simulink library "SAD"  (R2025b)
settings: Solver=VariableStepAuto  StartTime=0.0  StopTime=10.0  RelTol=1e-3
values from neighbouring files (symbols this model uses):
  c = astroConstants(5)*10^3    [RUN_ME.m]
  D = zeros(3)    [RUN_ME.m]
  Fe = 1358    [RUN_ME.m]
  I = [Ix 0 0; 0 Iy 0; 0 0 Iz]    [RUN_ME.m]
  Ix = (m_b/12)*((y_b^2)+(x_b^2))    (= 0.13)    [RUN_ME.m]
  Iy = (m_b/12)*((z_b^2)+(x_b^2))    (= 0.1)    [RUN_ME.m]
  Iz = (m_b/12)*((y_b^2)+(z_b^2))    (= 0.05)    [RUN_ME.m]
  n = sqrt(mu/a^3)    [RUN_ME.m]
  Ts = 0.1    [RUN_ME.m]
undefined symbols (not defined in the file or in its folder): A0, att0, Ir, Noise_pwr, Noise_st, omega_act_0, q0, RW_max_slope, RW_max_torque, RW_max_torque_descending_rate, RW_max_torque_start_descending, RW_min_torque, RW_offset, RW_tau_m, Satellite, w0, wr0
libraries: matrix_library x5, simulink x2, dspmathops x1
settings Model: Creator=ludod  LastModifiedBy=stefa

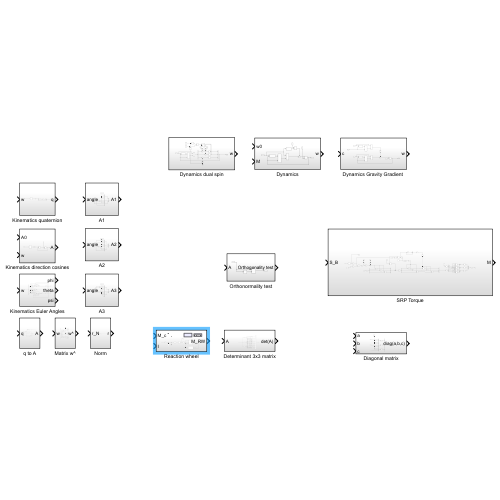
[thumbnail: Simulink's stored preview of the top-level diagram]
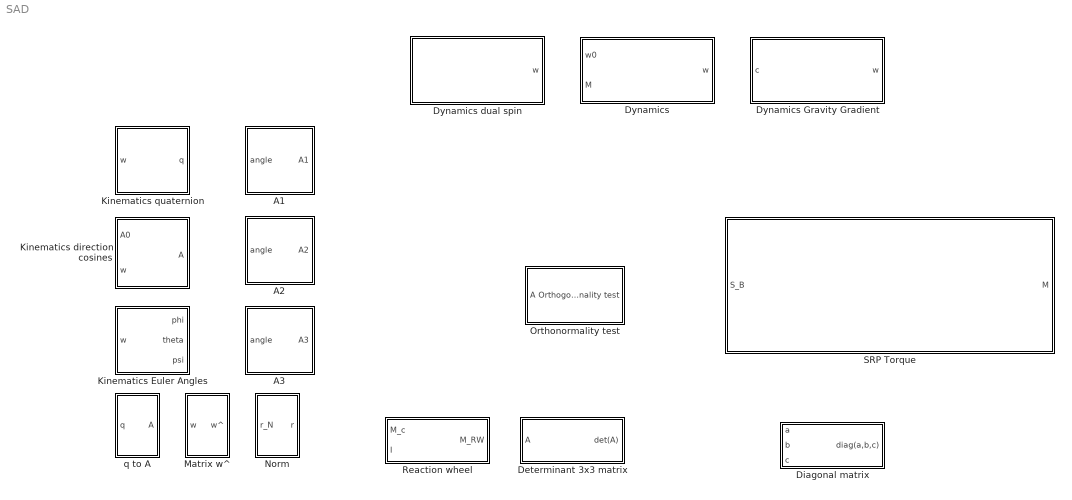
== system SAD ==
  A1 : Subsystem
  A2 : Subsystem
  A3 : Subsystem
  Determinant 3x3 matrix : Subsystem
  Diagonal matrix : Subsystem
  Dynamics : Subsystem
  "Dynamics Gravity Gradient " : Subsystem
  Dynamics dual spin : Subsystem
  Kinematics Euler Angles : Subsystem
  Kinematics direction cosines : Subsystem
  Kinematics quaternion : Subsystem
  Matrix w^ : Subsystem
  Norm : Subsystem
  Orthonormality test : Subsystem
  Reaction wheel : Subsystem
  SRP Torque : Subsystem
  q to A : Subsystem

== system SAD/A1 ==
  angle : Inport
  Cos : Trigonometry  Operator=cos
  Gain : Gain  Gain=-1
  Mux : Mux  Inputs=3
  Mux1 : Mux  Inputs=3
  Mux2 : Mux  Inputs=3
  One : Constant  OutDataTypeStr=Inherit: Inherit via back propagation
  Sin : Trigonometry
  Vector Concatenate : Concatenate  NumInputs=3  Mode=Multidimensional array  ConcatenateDimension=2
  Zero : Constant  Value=0  OutDataTypeStr=Inherit: Inherit via back propagation
  A1 : Outport
  wires:
  Zero/1 -> Mux2/1, Mux1/1, Mux/3, Mux/2
  One/1 -> Mux/1
  Sin/1 -> Mux2/2, Gain/1
  angle/1 -> Sin/1, Cos/1
  Vector Concatenate/1 -> A1/1  "A1"
  Gain/1 -> Mux1/3
  Cos/1 -> Mux2/3, Mux1/2
  Mux/1 -> Vector Concatenate/1
  Mux1/1 -> Vector Concatenate/2
  Mux2/1 -> Vector Concatenate/3

== system SAD/A2 ==
  angle : Inport
  Cos : Trigonometry  Operator=cos
  Gain : Gain  Gain=-1
  Mux : Mux  Inputs=3
  Mux1 : Mux  Inputs=3
  Mux2 : Mux  Inputs=3
  One : Constant  OutDataTypeStr=Inherit: Inherit via back propagation
  Sin : Trigonometry
  Vector Concatenate : Concatenate  NumInputs=3  Mode=Multidimensional array  ConcatenateDimension=2
  Zero : Constant  Value=0  OutDataTypeStr=Inherit: Inherit via back propagation
  A2 : Outport
  wires:
  Mux1/1 -> Vector Concatenate/2
  Mux2/1 -> Vector Concatenate/3
  Zero/1 -> Mux2/2, Mux1/3, Mux1/1, Mux/2
  One/1 -> Mux1/2
  Mux/1 -> Vector Concatenate/1
  Sin/1 -> Mux/3, Gain/1
  angle/1 -> Sin/1, Cos/1
  Vector Concatenate/1 -> A2/1  "A2"
  Cos/1 -> Mux2/3, Mux/1
  Gain/1 -> Mux2/1

== system SAD/A3 ==
  angle : Inport
  Cos : Trigonometry  Operator=cos
  Gain : Gain  Gain=-1
  Mux : Mux  Inputs=3
  Mux1 : Mux  Inputs=3
  Mux2 : Mux  Inputs=3
  One : Constant  OutDataTypeStr=Inherit: Inherit via back propagation
  Sin : Trigonometry
  Vector Concatenate : Concatenate  NumInputs=3  Mode=Multidimensional array  ConcatenateDimension=2
  Zero : Constant  Value=0  OutDataTypeStr=Inherit: Inherit via back propagation
  A3 : Outport
  wires:
  Mux1/1 -> Vector Concatenate/2
  Mux2/1 -> Vector Concatenate/3
  Zero/1 -> Mux1/3, Mux2/2, Mux2/1, Mux/3
  Mux/1 -> Vector Concatenate/1
  Sin/1 -> Mux1/1, Gain/1
  angle/1 -> Sin/1, Cos/1
  Vector Concatenate/1 -> A3/1  "A3"
  Cos/1 -> Mux1/2, Mux/1
  Gain/1 -> Mux/2
  One/1 -> Mux2/3

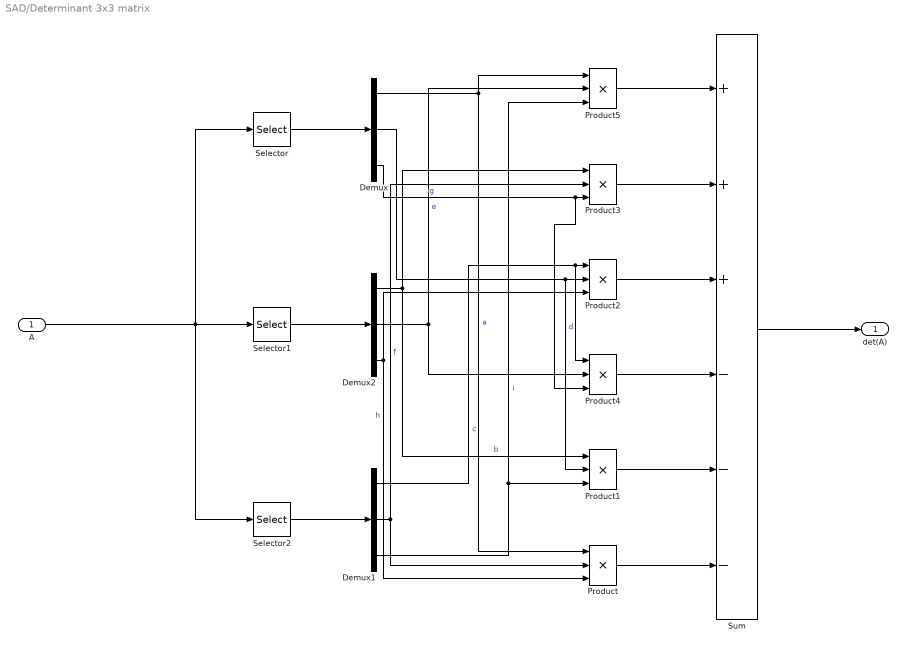
== system SAD/Determinant 3x3 matrix ==
  A : Inport
  Demux : Demux  Outputs=3
  Demux1 : Demux  Outputs=3
  Demux2 : Demux  Outputs=3
  Product{,1..5} (6 alike) : Product  Inputs=3
  Selector : Selector  NumberOfDimensions=2  InputPortWidth=3  IndexOptions=Index vector (dialog),Index vector (dialog)  Indices=1:3,1  OutputSizes=1,1
  Selector1 : Selector  NumberOfDimensions=2  InputPortWidth=3  IndexOptions=Index vector (dialog),Index vector (dialog)  Indices=1:3,2  OutputSizes=1,1
  Selector2 : Selector  NumberOfDimensions=2  InputPortWidth=3  IndexOptions=Index vector (dialog),Index vector (dialog)  Indices=1:3,3  OutputSizes=1,1
  Sum : Sum  Inputs=+++---
  det(A) : Outport
  wires:
  A/1 -> Selector1/1, Selector/1, Selector2/1
  Selector/1 -> Demux/1
  Selector1/1 -> Demux2/1
  Selector2/1 -> Demux1/1
  Demux/1 -> Product/1, Product5/1  "a"
  Demux/2 -> Product2/2, Product1/2  "d"
  Demux/3 -> Product4/3, Product3/3  "g"
  Demux2/1 -> Product1/1, Product3/1  "b"
  Demux2/2 -> Product4/2, Product5/2  "e"
  Demux2/3 -> Product2/3, Product/3  "h"
  Demux1/1 -> Product4/1, Product2/1  "c"
  Demux1/2 -> Product/2, Product3/2  "f"
  Demux1/3 -> Product1/3, Product5/3  "i"
  Product/1 -> Sum/6
  Product1/1 -> Sum/5
  Product4/1 -> Sum/4
  Product2/1 -> Sum/3
  Product3/1 -> Sum/2
  Product5/1 -> Sum/1
  Sum/1 -> det(A)/1

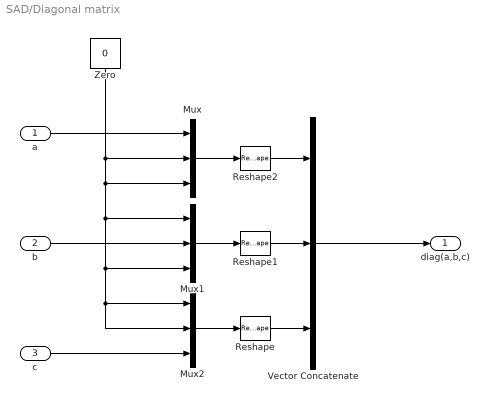
== system SAD/Diagonal matrix ==
  a : Inport
  b : Inport  Port=2
  c : Inport  Port=3
  Mux : Mux  Inputs=3
  Mux1 : Mux  Inputs=3
  Mux2 : Mux  Inputs=3
  Reshape : Reshape  OutputDimensionality=Column vector (2-D)
  Reshape1 : Reshape  OutputDimensionality=Column vector (2-D)
  Reshape2 : Reshape  OutputDimensionality=Column vector (2-D)
  Vector Concatenate : Concatenate  NumInputs=3  Mode=Multidimensional array  ConcatenateDimension=2
  Zero : Constant  Value=0  OutDataTypeStr=Inherit: Inherit via back propagation
  diag(a,b,c) : Outport
  wires:
  a/1 -> Mux/1
  b/1 -> Mux1/2
  c/1 -> Mux2/3
  Zero/1 -> Mux/2, Mux/3, Mux1/1, Mux1/3, Mux2/2, Mux2/1
  Mux/1 -> Reshape2/1
  Mux1/1 -> Reshape1/1
  Mux2/1 -> Reshape/1
  Vector Concatenate/1 -> diag(a,b,c)/1
  Reshape2/1 -> Vector Concatenate/1
  Reshape1/1 -> Vector Concatenate/2
  Reshape/1 -> Vector Concatenate/3

== system SAD/Dynamics ==
  w0 : Inport
  M : Inport  Port=2
  Constant : Constant  Value=I
  Cross Product : matrix_library/Cross Product
  Divide : Product  Inputs=*/
  Extract Diagonal : matrix_library/Extract Diagonal
      settings: LibrarySourceBlock=|
      | simulink/Matrix
      | Operations/Extract Diagonal
  Integrator : Integrator  InitialConditionSource=external
  Product : Product  Multiplication=Matrix(*)
  Product1 : Product  Inputs=/*  Multiplication=Matrix(*)
  Sum : Sum  Inputs=++|
  w : Outport
  wires:
  w0/1 -> Integrator/2
  Constant/1 -> Product1/1, Extract Diagonal/1, Product/1
  Integrator/1 -> w/1, Product/2, Cross Product/2
  Cross Product/1 -> Product1/2
  Product/1 -> Cross Product/1
  M/1 -> Divide/1
  Divide/1 -> Sum/1
  Product1/1 -> Sum/2
  Sum/1 -> Integrator/1
  Extract Diagonal/1 -> Divide/2

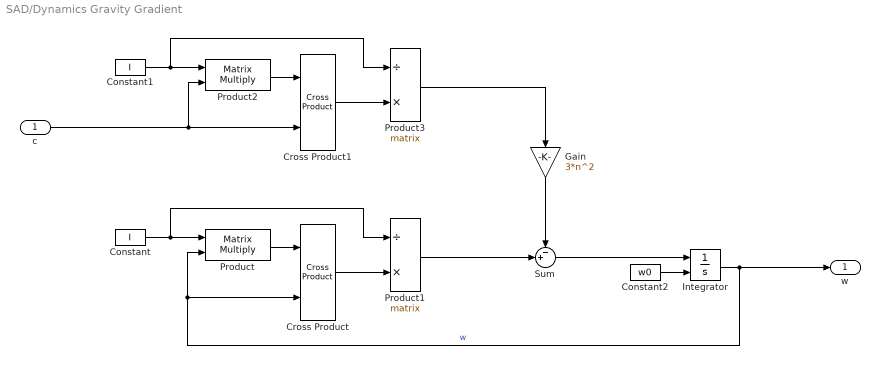
== system SAD/Dynamics Gravity Gradient  ==
  c : Inport
  Constant : Constant  Value=I
  Constant1 : Constant  Value=I
  Constant2 : Constant  Value=w0
  Cross Product : matrix_library/Cross Product
  Cross Product1 : matrix_library/Cross Product
  Gain : Gain  Gain=3*n^2
  Integrator : Integrator  InitialConditionSource=external
  Product : Product  Multiplication=Matrix(*)
  Product1 : Product  Inputs=/*  Multiplication=Matrix(*)
  Product2 : Product  Multiplication=Matrix(*)
  Product3 : Product  Inputs=/*  Multiplication=Matrix(*)
  Sum : Sum  Inputs=-+|
  w : Outport
  wires:
  Product/1 -> Cross Product/1
  Product2/1 -> Cross Product1/1
  Integrator/1 -> w/1, Cross Product/2, Product/2  "w"
  Product3/1 -> Gain/1
  c/1 -> Product2/2, Cross Product1/2
  Constant2/1 -> Integrator/2
  Constant1/1 -> Product3/1, Product2/1
  Cross Product/1 -> Product1/2
  Product1/1 -> Sum/2
  Sum/1 -> Integrator/1
  Constant/1 -> Product/1, Product1/1
  Gain/1 -> Sum/1
  Cross Product1/1 -> Product3/2

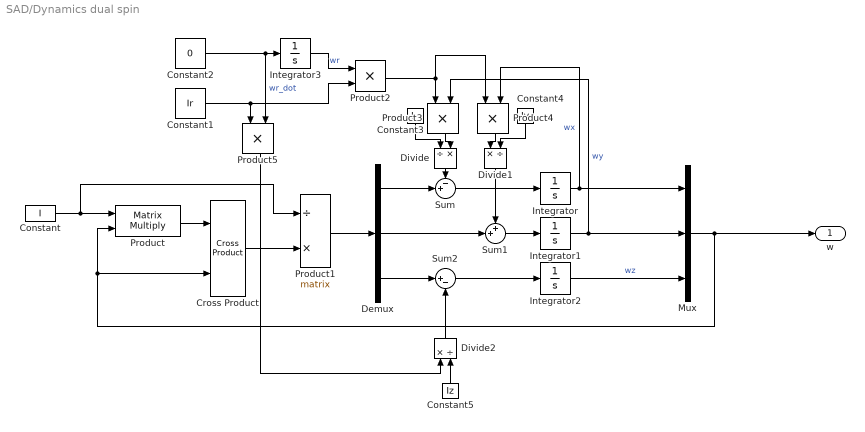
== system SAD/Dynamics dual spin ==
  Constant : Constant  Value=I
  Constant1 : Constant  Value=Ir
  Constant2 : Constant  Value=0
  Constant3 : Constant  Value=Ix
  Constant4 : Constant  Value=Iy
  Constant5 : Constant  Value=Iz
  Cross Product : matrix_library/Cross Product
  Demux : Demux  Outputs=3
  Divide : Product  Inputs=/*
  Divide1 : Product  Inputs=*/
  Divide2 : Product  Inputs=*/
  Integrator : Integrator  InitialCondition=w0(1)
  Integrator1 : Integrator  InitialCondition=w0(2)
  Integrator2 : Integrator  InitialCondition=w0(3)
  Integrator3 : Integrator  InitialCondition=wr0
  Mux : Mux  Inputs=3
  Product : Product  Multiplication=Matrix(*)
  Product1 : Product  Inputs=/*  Multiplication=Matrix(*)
  Product{2..5} (4 alike) : Product
  Sum : Sum  Inputs=-+|
  Sum1 : Sum  Inputs=++|
  Sum2 : Sum  Inputs=|+-
  w : Outport
  wires:
  Constant1/1 -> Product2/2, Product5/1
  Product5/1 -> Divide2/1
  Divide2/1 -> Sum2/2
  Integrator1/1 -> Mux/2, Product3/2  "wy"
  Demux/2 -> Sum1/2
  Cross Product/1 -> Product1/2
  Demux/3 -> Sum2/1
  Sum/1 -> Integrator/1
  Divide/1 -> Sum/1
  Constant/1 -> Product1/1, Product/1
  Mux/1 -> w/1, Product/2, Cross Product/2
  Constant4/1 -> Divide1/2
  Demux/1 -> Sum/2
  Sum1/1 -> Integrator1/1
  Integrator/1 -> Mux/1, Product4/2  "wx"
  Integrator2/1 -> Mux/3  "wz"
  Product/1 -> Cross Product/1
  Product4/1 -> Divide1/1
  Product2/1 -> Product4/1, Product3/1
  Constant3/1 -> Divide/1
  Constant2/1 -> Product5/2, Integrator3/1  "wr_dot"
  Product3/1 -> Divide/2
  Product1/1 -> Demux/1
  Constant5/1 -> Divide2/2
  Integrator3/1 -> Product2/1  "wr"
  Sum2/1 -> Integrator2/1
  Divide1/1 -> Sum1/1

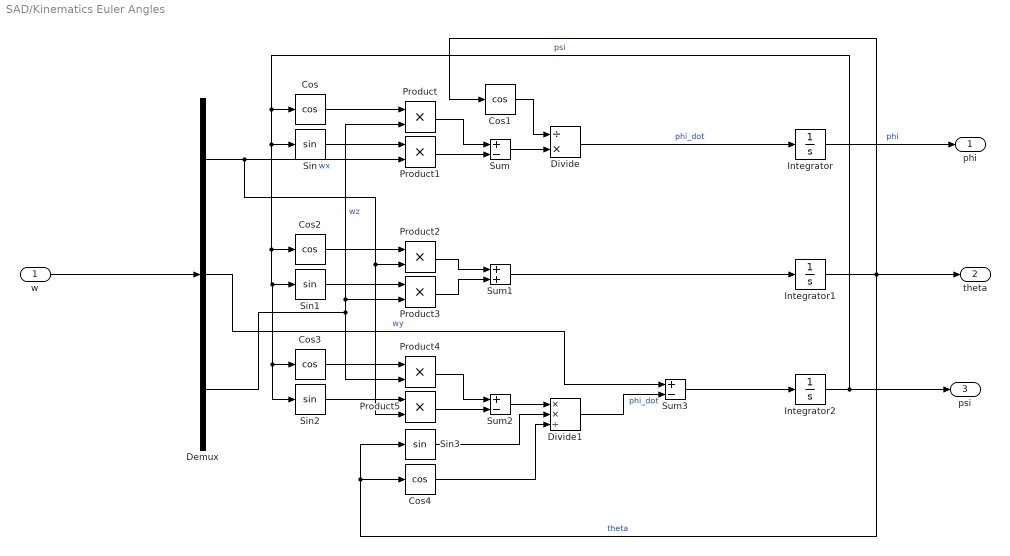
== system SAD/Kinematics Euler Angles ==
  w : Inport
  Cos{,1..4} (5 alike) : Trigonometry  Operator=cos
  Demux : Demux  Outputs=3
  Divide : Product  Inputs=/*
  Divide1 : Product  Inputs=**/
  Integrator : Integrator  InitialCondition=att0(1)  WrapState=on
  Integrator1 : Integrator  InitialCondition=att0(2)  WrapState=on
  Integrator2 : Integrator  InitialCondition=att0(3)  WrapState=on
  Product{,1..5} (6 alike) : Product
  Sin{,1..3} (4 alike) : Trigonometry
  Sum : Sum  Inputs=+-
  Sum1 : Sum
  Sum2 : Sum  Inputs=+-
  Sum3 : Sum  Inputs=+-
  phi : Outport
  theta : Outport  Port=2
  psi : Outport  Port=3
  wires:
  Cos1/1 -> Divide/1
  Demux/3 -> Product4/2, Product3/2, Product/2  "wz"
  Sin3/1 -> Divide1/2
  Product2/1 -> Sum1/1
  Product/1 -> Sum/1
  Integrator2/1 -> psi/1, Sin2/1, Cos3/1, Sin1/1, Cos2/1, Sin/1, Cos/1  "psi"
  Sin1/1 -> Product3/1
  Sin/1 -> Product1/1
  Integrator1/1 -> theta/1, Cos4/1, Sin3/1, Cos1/1  "theta"
  Cos2/1 -> Product2/1
  Cos/1 -> Product/1
  Sum1/1 -> Integrator1/1
  Cos3/1 -> Product4/1
  Demux/1 -> Product1/2, Product5/2, Product2/2  "wx"
  Integrator/1 -> phi/1  "phi"
  Product4/1 -> Sum2/1
  Sin2/1 -> Product5/1
  Product3/1 -> Sum1/2
  Demux/2 -> Sum3/1  "wy"
  Product1/1 -> Sum/2
  Sum/1 -> Divide/2
  Divide/1 -> Integrator/1  "phi_dot"
  Product5/1 -> Sum2/2
  Sum2/1 -> Divide1/1
  w/1 -> Demux/1
  Sum3/1 -> Integrator2/1
  Divide1/1 -> Sum3/2  "phi_dot"
  Cos4/1 -> Divide1/3

== system SAD/Kinematics direction cosines ==
  A0 : Inport
  w : Inport  Port=2
  Gain : Gain  Gain=-1
  Integrator : Integrator  InitialConditionSource=external  InitialCondition=A0
  Matrix w^ : Subsystem
  Product1 : Product  Multiplication=Matrix(*)
  A : Outport
  wires:
  Product1/1 -> Integrator/1  "A_dot"
  Matrix w^/1(w^) -> Gain/1  "w^"
  Integrator/1 -> A/1, Product1/2  "A"
  Gain/1 -> Product1/1
  w/1 -> Matrix w^/1(w)
  A0/1 -> Integrator/2

== system SAD/Kinematics quaternion ==
  w : Inport
  Gain : Gain  Gain=1/2
  Integrator1 : Integrator  InitialCondition=q0
  Omega matrix : Subsystem
  Product : Product  Multiplication=Matrix(*)
  Reshape : Reshape  OutputDimensionality=Column vector (2-D)
  q : Outport
  wires:
  Reshape/1 -> q/1, Product/2
  Integrator1/1 -> Reshape/1  "q"
  Omega matrix/1(Omega) -> Gain/1
  w/1 -> Omega matrix/1(w)
  Product/1 -> Integrator1/1  "q_dot"
  Gain/1 -> Product/1

== system SAD/Matrix w^ ==
  w : Inport
  Demux1 : Demux  Outputs=3
  Gain : Gain  Gain=-1
  Gain3 : Gain  Gain=-1
  Gain5 : Gain  Gain=-1
  Mux : Mux  Inputs=3
  Mux1 : Mux  Inputs=3
  Mux2 : Mux  Inputs=3
  Vector Concatenate : Concatenate  NumInputs=3  Mode=Multidimensional array  ConcatenateDimension=2
  Zero : Constant  Value=0  OutDataTypeStr=Inherit: Inherit via back propagation
  w^ : Outport
  wires:
  Mux1/1 -> Vector Concatenate/3
  Vector Concatenate/1 -> w^/1
  Demux1/3 -> Mux/2, Gain3/1
  Demux1/1 -> Mux2/3, Gain5/1
  Demux1/2 -> Mux1/1, Gain/1
  w/1 -> Demux1/1
  Mux/1 -> Vector Concatenate/1
  Mux2/1 -> Vector Concatenate/2
  Gain/1 -> Mux/3
  Gain3/1 -> Mux2/1
  Gain5/1 -> Mux1/2
  Zero/1 -> Mux1/3, Mux2/2, Mux/1

== system SAD/Norm ==
  r_N : Inport
  MatrixMultiply : Product  Multiplication=Matrix(*)
  Square Root : Sqrt
  Transpose : Math  Operator=transpose
  r : Outport
  wires:
  MatrixMultiply/1 -> Square Root/1
  r_N/1 -> MatrixMultiply/2, Transpose/1
  Transpose/1 -> MatrixMultiply/1
  Square Root/1 -> r/1  "r"

== system SAD/Orthonormality test ==
  A : Inport
  Product2 : Product  Multiplication=Matrix(*)
  Transpose : Math  Operator=transpose
  Orthogonality test : Outport
  wires:
  Transpose/1 -> Product2/2
  A/1 -> Product2/1, Transpose/1
  Product2/1 -> Orthogonality test/1  "A_dot"

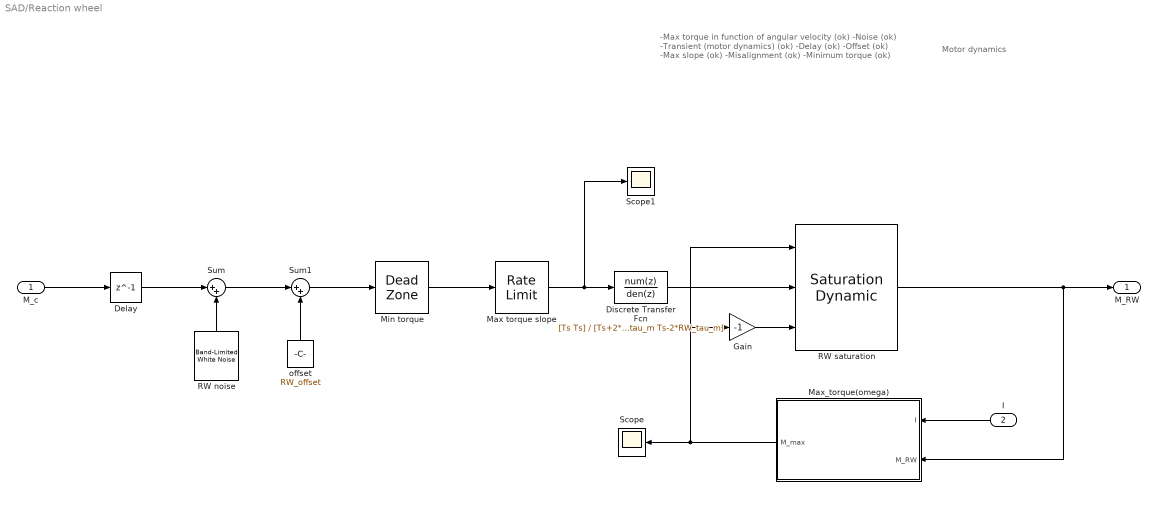
== system SAD/Reaction wheel ==
  note: Motor dynamics
  note: -Max torque in function of angular velocity (ok)
      | -Noise (ok)
      | -Transient (motor dynamics) (ok)
      | -Delay (ok)
      | -Offset (ok)
      | -Max slope (ok)
      | -Misalignment (ok)
      | -Minimum torque (ok)
  M_c : Inport
  I : Inport  Port=2
  Delay : Delay  DelayLength=1
  Discrete Transfer Fcn : DiscreteTransferFcn  Numerator=[Ts Ts]  Denominator=[Ts+2*RW_tau_m Ts-2*RW_tau_m]
  Gain : Gain  Gain=-1
  Max torque slope : RateLimiter  RisingSlewLimit=RW_max_slope  FallingSlewLimit=-RW_max_slope  SampleTimeMode=inherited
  Max_torque(omega) : Subsystem
  Min torque : DeadZone  LowerValue=-RW_min_torque  UpperValue=RW_min_torque
  RW noise : simulink/Sources/Band-Limited White Noise  Cov=[Noise_pwr]  Ts=Noise_st  seed=[23341]
  RW saturation : simulink/Discontinuities/Saturation Dynamic  OutMin=[]  OutMax=[]  OutDataTypeStr=Inherit: Same as second input  OutDataType=fixdt(1, 16)  OutScaling=2^-10  DoSatur=off
  Scope : Scope
  Scope1 : Scope
      settings: DataLoggingVariableName=ScopeData2
  Sum : Sum  Inputs=|++
  Sum1 : Sum  Inputs=|++
  offset : Constant  Value=RW_offset
  M_RW : Outport
  wires:
  M_c/1 -> Delay/1
  Gain/1 -> RW saturation/3
  RW saturation/1 -> Max_torque(omega)/2(M_RW), M_RW/1
  RW noise/1 -> Sum/2
  Sum/1 -> Sum1/1
  offset/1 -> Sum1/2
  Sum1/1 -> Min torque/1
  Max_torque(omega)/1(M_max) -> Gain/1, RW saturation/1, Scope/1
  I/1 -> Max_torque(omega)/1(I)
  Delay/1 -> Sum/1
  Min torque/1 -> Max torque slope/1
  Max torque slope/1 -> Discrete Transfer Fcn/1, Scope1/1
  Discrete Transfer Fcn/1 -> RW saturation/2

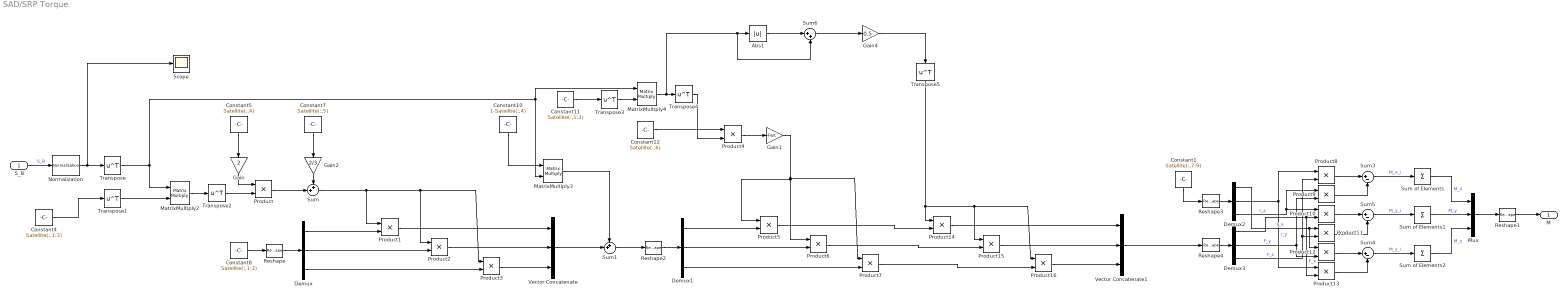
== system SAD/SRP Torque ==
  S_B : Inport
  Abs1 : Abs  SaturateOnIntegerOverflow=off
  Constant1 : Constant  Value=Satellite(:,7:9)  VectorParams1D=off
  Constant10 : Constant  Value=1-Satellite(:,4)  VectorParams1D=off
  Constant11 : Constant  Value=Satellite(:,1:3)  VectorParams1D=off
  Constant12 : Constant  Value=Satellite(:,6)  VectorParams1D=off
  Constant4 : Constant  Value=Satellite(:,1:3)
  Constant5 : Constant  Value=Satellite(:,4)  VectorParams1D=off
  Constant7 : Constant  Value=Satellite(:,5)  VectorParams1D=off
  Constant8 : Constant  Value=Satellite(:,1:3)
  Demux{,1..3} (4 alike) : Demux  Outputs=3
  Gain : Gain  Gain=2
  Gain1 : Gain  Gain=-Fe/c
  Gain2 : Gain  Gain=2/3
  Gain4 : Gain  Gain=0.5
  MatrixMultiply2 : Product  Multiplication=Matrix(*)
  MatrixMultiply3 : Product  Multiplication=Matrix(*)
  MatrixMultiply4 : Product  Multiplication=Matrix(*)
  Mux : Mux  Inputs=3
  Normalization : dspmathops/Normalization  NormType=2-norm  Bias=1e-10  NormOver=Each column  Dimension=1  roundingMode=Floor  overflowMode=off  accumDataTypeStr=Inherit: Same as product output  accumLastDataTypeStr=Inherit: Same as product output  outputDataTypeStr=Inherit: Same as product output  outputMin=[]  outputMax=[]  outputLastDataTypeStr=Inherit: Same as product output
  Product{,1..16} (17 alike) : Product
  Reshape{,1..4} (5 alike) : Reshape  OutputDimensionality=Column vector (2-D)
  Scope : Scope
      settings: ActiveDisplayYMinimum=-1  ActiveDisplayYMaximum=1  DataLoggingVariableName=ScopeData3
  Sum : Sum  Inputs=++|
  Sum of Elements : Sum  Inputs=+
  Sum of Elements1 : Sum  Inputs=+
  Sum of Elements2 : Sum  Inputs=+
  Sum1 : Sum  Inputs=++|
  Sum3 : Sum  Inputs=|+-
  Sum4 : Sum  Inputs=|+-
  Sum5 : Sum  Inputs=|+-
  Sum6 : Sum  Inputs=|++
  Transpose{,1..5} (6 alike) : Math  Operator=transpose
  Vector Concatenate : Concatenate  NumInputs=3  Mode=Multidimensional array  ConcatenateDimension=2
  Vector Concatenate1 : Concatenate  NumInputs=3  Mode=Multidimensional array  ConcatenateDimension=2
  M : Outport
  wires:
  Product4/1 -> Gain1/1
  Gain1/1 -> Product6/1, Product5/1, Product7/1
  Vector Concatenate/1 -> Sum1/2
  Product/1 -> Sum/2
  Transpose/1 -> MatrixMultiply4/1, MatrixMultiply3/2, MatrixMultiply2/1
  Gain/1 -> Product/1
  Sum/1 -> Product1/1, Product2/1, Product3/1
  MatrixMultiply3/1 -> Sum1/1
  Gain2/1 -> Sum/1
  Constant4/1 -> Transpose1/1
  MatrixMultiply2/1 -> Transpose2/1
  Constant11/1 -> Transpose3/1
  S_B/1 -> Normalization/1  "S_B"
  Demux/2 -> Product2/2
  Demux/3 -> Product3/2
  Constant5/1 -> Gain/1
  Transpose2/1 -> Product/2
  Transpose1/1 -> MatrixMultiply2/2
  Constant7/1 -> Gain2/1
  Reshape/1 -> Demux/1
  Demux1/3 -> Product7/2
  Demux/1 -> Product1/2
  Product2/1 -> Vector Concatenate/2
  Constant8/1 -> Reshape/1
  Product1/1 -> Vector Concatenate/1
  Product3/1 -> Vector Concatenate/3
  Sum1/1 -> Reshape2/1
  Constant10/1 -> MatrixMultiply3/1
  Demux1/2 -> Product6/2
  Demux1/1 -> Product5/2
  Reshape2/1 -> Demux1/1
  Constant12/1 -> Product4/1
  Normalization/1 -> Scope/1, Transpose/1
  Constant1/1 -> Reshape3/1
  Vector Concatenate1/1 -> Reshape4/1
  Demux2/1 -> Product12/1, Product11/1  "r_x"
  Demux2/2 -> Product8/1, Product13/1  "r_y"
  Demux2/3 -> Product10/1, Product9/1  "r_z"
  Demux3/1 -> Product10/2, Product13/2  "F_x"
  Demux3/2 -> Product12/2, Product9/2  "F_y"
  Demux3/3 -> Product11/2, Product8/2  "F_z"
  Reshape3/1 -> Demux2/1
  Reshape4/1 -> Demux3/1
  Product12/1 -> Sum4/1
  Product10/1 -> Sum5/1
  Product8/1 -> Sum3/1
  Product9/1 -> Sum3/2
  Product11/1 -> Sum5/2
  Product13/1 -> Sum4/2
  Sum3/1 -> Sum of Elements/1  "M_x_i"
  Sum5/1 -> Sum of Elements1/1  "M_y_i"
  Sum4/1 -> Sum of Elements2/1  "M_z_i"
  Sum of Elements/1 -> Mux/1  "M_x"
  Sum of Elements1/1 -> Mux/2  "M_y"
  Sum of Elements2/1 -> Mux/3  "M_z"
  Mux/1 -> Reshape1/1
  Reshape1/1 -> M/1
  Transpose3/1 -> MatrixMultiply4/2
  Transpose4/1 -> Product4/2
  Gain4/1 -> Transpose5/1
  MatrixMultiply4/1 -> Sum6/2, Abs1/1, Transpose4/1
  Abs1/1 -> Sum6/1
  Sum6/1 -> Gain4/1
  Transpose5/1 -> Product14/1, Product15/1, Product16/1
  Product5/1 -> Product14/2
  Product6/1 -> Product15/2
  Product7/1 -> Product16/2
  Product14/1 -> Vector Concatenate1/1
  Product15/1 -> Vector Concatenate1/2
  Product16/1 -> Vector Concatenate1/3

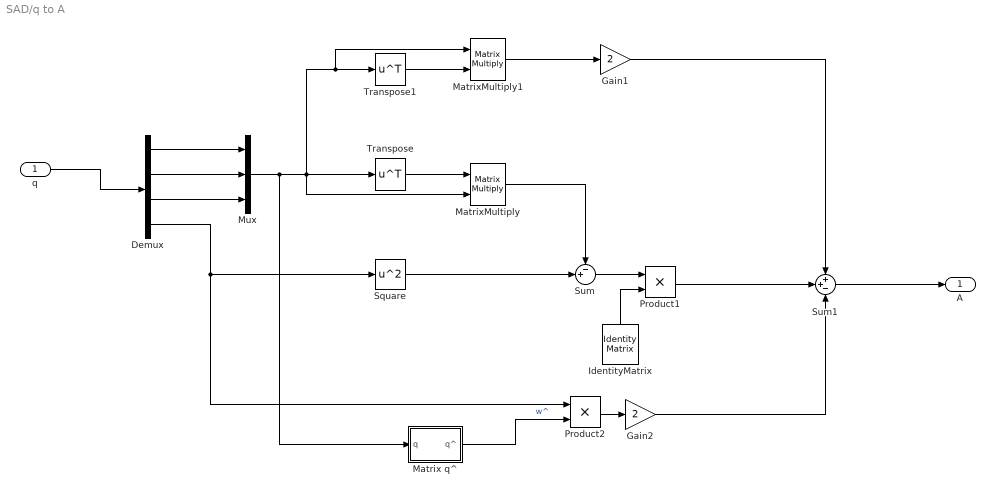
== system SAD/q to A ==
  q : Inport
  Demux : Demux
  Gain1 : Gain  Gain=2
  Gain2 : Gain  Gain=2
  IdentityMatrix : IdentityMatrix  OutputDimensions=3
  Matrix q^ : Subsystem
  MatrixMultiply : Product  Multiplication=Matrix(*)
  MatrixMultiply1 : Product  Multiplication=Matrix(*)
  Mux : Mux  Inputs=3
  Product1 : Product
  Product2 : Product
  Square : Math  Operator=square
  Sum : Sum  Inputs=-+|
  Sum1 : Sum  Inputs=++-
  Transpose : Math  Operator=transpose
  Transpose1 : Math  Operator=transpose
  A : Outport
  wires:
  Demux/2 -> Mux/2
  Sum1/1 -> A/1
  q/1 -> Demux/1
  Demux/1 -> Mux/1
  Demux/3 -> Mux/3
  IdentityMatrix/1 -> Product1/2
  MatrixMultiply1/1 -> Gain1/1
  Transpose1/1 -> MatrixMultiply1/2
  Gain1/1 -> Sum1/1
  MatrixMultiply/1 -> Sum/1
  Transpose/1 -> MatrixMultiply/1
  Mux/1 -> Matrix q^/1(q), Transpose/1, MatrixMultiply1/1, Transpose1/1, MatrixMultiply/2
  Demux/4 -> Product2/1, Square/1
  Matrix q^/1(q^) -> Product2/2  "w^"
  Gain2/1 -> Sum1/3
  Product2/1 -> Gain2/1
  Square/1 -> Sum/2
  Sum/1 -> Product1/1
  Product1/1 -> Sum1/2

== system SAD/Kinematics direction cosines/Matrix w^ ==
  w : Inport
  Demux1 : Demux  Outputs=3
  Gain : Gain  Gain=-1
  Gain3 : Gain  Gain=-1
  Gain5 : Gain  Gain=-1
  Mux : Mux  Inputs=3
  Mux1 : Mux  Inputs=3
  Mux2 : Mux  Inputs=3
  Vector Concatenate : Concatenate  NumInputs=3  Mode=Multidimensional array  ConcatenateDimension=2
  Zero : Constant  Value=0  OutDataTypeStr=Inherit: Inherit via back propagation
  w^ : Outport
  wires:
  Mux1/1 -> Vector Concatenate/3
  Vector Concatenate/1 -> w^/1
  Demux1/3 -> Mux/2, Gain3/1
  Demux1/1 -> Mux2/3, Gain5/1
  Demux1/2 -> Mux1/1, Gain/1
  w/1 -> Demux1/1
  Mux/1 -> Vector Concatenate/1
  Mux2/1 -> Vector Concatenate/2
  Gain/1 -> Mux/3
  Gain3/1 -> Mux2/1
  Gain5/1 -> Mux1/2
  Zero/1 -> Mux1/3, Mux2/2, Mux/1

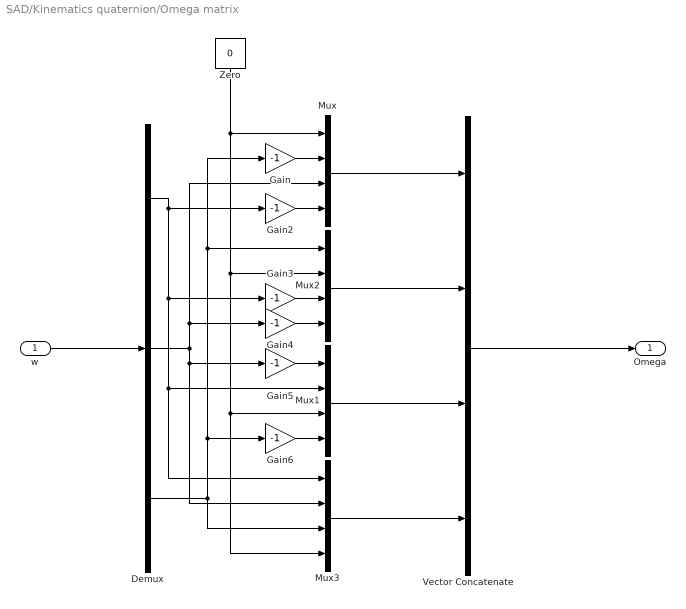
== system SAD/Kinematics quaternion/Omega matrix ==
  w : Inport
  Demux : Demux  Outputs=3
  Gain{,2..6} (6 alike) : Gain  Gain=-1
  Mux{,1..3} (4 alike) : Mux
  Vector Concatenate : Concatenate  NumInputs=4  Mode=Multidimensional array  ConcatenateDimension=2
  Zero : Constant  Value=0  OutDataTypeStr=Inherit: Inherit via back propagation
  Omega : Outport
  wires:
  Demux/2 -> Mux3/2, Gain5/1, Gain4/1, Mux/3
  Gain3/1 -> Mux2/3
  Demux/1 -> Mux1/2, Mux3/1, Gain3/1, Gain2/1
  Demux/3 -> Mux3/3, Gain6/1, Mux2/1, Gain/1
  Gain5/1 -> Mux1/1
  w/1 -> Demux/1
  Gain/1 -> Mux/2
  Vector Concatenate/1 -> Omega/1
  Zero/1 -> Mux/1, Mux2/2, Mux1/3, Mux3/4
  Mux1/1 -> Vector Concatenate/3
  Gain6/1 -> Mux1/4
  Mux/1 -> Vector Concatenate/1
  Mux2/1 -> Vector Concatenate/2
  Mux3/1 -> Vector Concatenate/4
  Gain2/1 -> Mux/4
  Gain4/1 -> Mux2/4

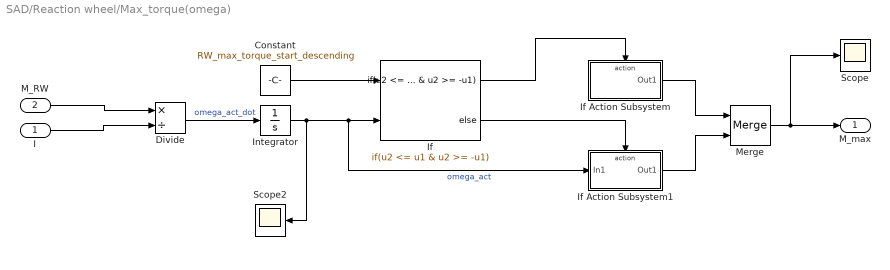
== system SAD/Reaction wheel/Max_torque(omega) ==
  I : Inport
  M_RW : Inport  Port=2
  Constant : Constant  Value=RW_max_torque_start_descending
  Divide : Product  Inputs=*/
  If : If  NumInputs=2  IfExpression=u2 <= u1 & u2 >= -u1
  If Action Subsystem : Subsystem  TreatAsAtomicUnit=on
  If Action Subsystem1 : Subsystem  TreatAsAtomicUnit=on
  Integrator : Integrator  InitialCondition=omega_act_0
  Merge : Merge
  Scope : Scope
      settings: ActiveDisplayYMinimum=0.99988609158163688  ActiveDisplayYMaximum=1.0001616250891987
  Scope2 : Scope
      settings: ActiveDisplayYMinimum=-55.538061989690384  ActiveDisplayYMaximum=499.84255790721357  DataLoggingVariableName=ScopeData4
  M_max : Outport
  wires:
  M_RW/1 -> Divide/1
  If Action Subsystem/1(Out1) -> Merge/1
  If/2 -> If Action Subsystem1/Action
  If Action Subsystem1/1(Out1) -> Merge/2
  Integrator/1 -> Scope2/1, If/2, If Action Subsystem1/1(In1)  "omega_act"
  Merge/1 -> M_max/1, Scope/1
  If/1 -> If Action Subsystem/Action
  Divide/1 -> Integrator/1  "omega_act_dot"
  Constant/1 -> If/1
  I/1 -> Divide/2

== system SAD/q to A/Matrix q^ ==
  q : Inport
  Demux1 : Demux  Outputs=3
  Gain : Gain  Gain=-1
  Gain3 : Gain  Gain=-1
  Gain5 : Gain  Gain=-1
  Mux : Mux  Inputs=3
  Mux1 : Mux  Inputs=3
  Mux2 : Mux  Inputs=3
  Vector Concatenate : Concatenate  NumInputs=3  Mode=Multidimensional array  ConcatenateDimension=2
  Zero : Constant  Value=0  OutDataTypeStr=Inherit: Inherit via back propagation
  q^ : Outport
  wires:
  Mux1/1 -> Vector Concatenate/3
  Vector Concatenate/1 -> q^/1
  Demux1/3 -> Mux/2, Gain3/1
  Demux1/1 -> Mux2/3, Gain5/1
  Demux1/2 -> Mux1/1, Gain/1
  q/1 -> Demux1/1
  Mux/1 -> Vector Concatenate/1
  Mux2/1 -> Vector Concatenate/2
  Gain/1 -> Mux/3
  Gain3/1 -> Mux2/1
  Gain5/1 -> Mux1/2
  Zero/1 -> Mux1/3, Mux2/2, Mux/1

== system SAD/Reaction wheel/Max_torque(omega)/If Action Subsystem ==
  Action Port : ActionPort
  Constant : Constant  Value=RW_max_torque
  Out1 : Outport
  wires:
  Constant/1 -> Out1/1

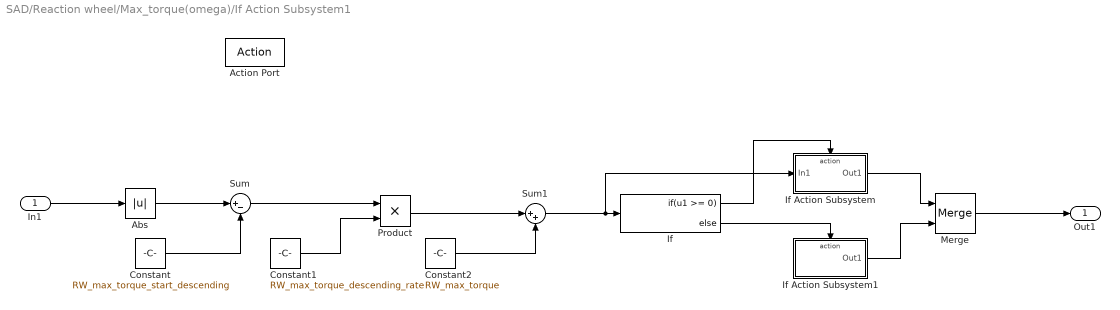
== system SAD/Reaction wheel/Max_torque(omega)/If Action Subsystem1 ==
  In1 : Inport
  Action Port : ActionPort
  Abs : Abs  SaturateOnIntegerOverflow=off
  Constant : Constant  Value=RW_max_torque_start_descending
  Constant1 : Constant  Value=RW_max_torque_descending_rate
  Constant2 : Constant  Value=RW_max_torque
  If : If  IfExpression=u1 >= 0
  If Action Subsystem : Subsystem  TreatAsAtomicUnit=on
  If Action Subsystem1 : Subsystem  TreatAsAtomicUnit=on
  Merge : Merge
  Product : Product
  Sum : Sum  Inputs=|+-
  Sum1 : Sum  Inputs=|++
  Out1 : Outport
  wires:
  In1/1 -> Abs/1
  Constant/1 -> Sum/2
  Sum/1 -> Product/1
  Constant1/1 -> Product/2
  Product/1 -> Sum1/1
  Constant2/1 -> Sum1/2
  Sum1/1 -> If Action Subsystem/1(In1), If/1
  If/1 -> If Action Subsystem/Action
  If/2 -> If Action Subsystem1/Action
  Merge/1 -> Out1/1
  If Action Subsystem1/1(Out1) -> Merge/2
  If Action Subsystem/1(Out1) -> Merge/1
  Abs/1 -> Sum/1

== system SAD/Reaction wheel/Max_torque(omega)/If Action Subsystem1/If Action Subsystem ==
  In1 : Inport
  Action Port : ActionPort
  Out1 : Outport
  wires:
  In1/1 -> Out1/1

== system SAD/Reaction wheel/Max_torque(omega)/If Action Subsystem1/If Action Subsystem1 ==
  Action Port : ActionPort
  Zero : Constant  Value=0  OutDataTypeStr=Inherit: Inherit via back propagation
  Out1 : Outport
  wires:
  Zero/1 -> Out1/1
